simulink model "Question2"  (R2023b)
settings: Solver=VariableStepAuto  StartTime=0.0  StopTime=10.0  RelTol=1e-3
libraries: simulink x1
settings Model: Creator=joaquinsalas  LastModifiedBy=joaquinsalas

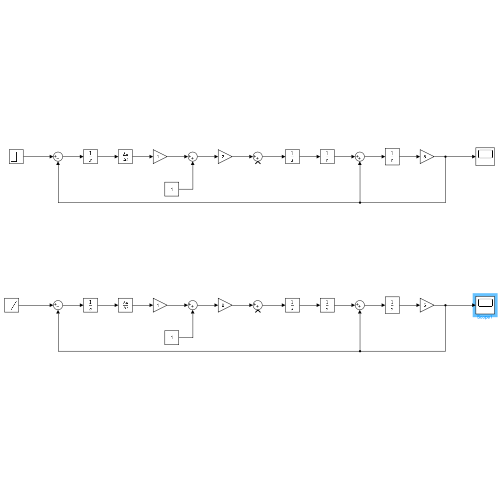
[thumbnail: Simulink's stored preview of the top-level diagram]
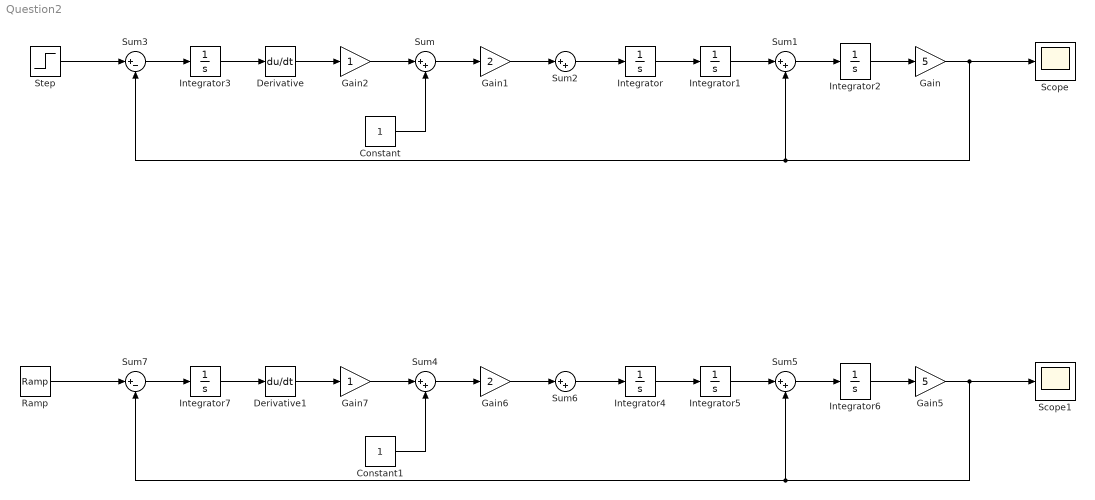
== system Question2 ==
  Constant : Constant
  Constant1 : Constant
  Derivative : Derivative
  Derivative1 : Derivative
  Gain : Gain  Gain=5
  Gain1 : Gain  Gain=2
  Gain2 : Gain
  Gain5 : Gain  Gain=5
  Gain6 : Gain  Gain=2
  Gain7 : Gain
  Integrator{,1..7} (8 alike) : Integrator
  Ramp : simulink/Sources/Ramp  slope=1  start=0  InitialOutput=0
  Scope : Scope
  Scope1 : Scope
  Step : Step  SampleTime=0
  Sum{,1..2,4..6} (6 alike) : Sum  Inputs=|++
  Sum3 : Sum  Inputs=|+-
  Sum7 : Sum  Inputs=|+-
  wires:
  Integrator/1 -> Integrator1/1
  Integrator2/1 -> Gain/1
  Integrator1/1 -> Sum1/1
  Sum1/1 -> Integrator2/1
  Integrator3/1 -> Derivative/1
  Constant/1 -> Sum/2
  Gain2/1 -> Sum/1
  Derivative/1 -> Gain2/1
  Sum/1 -> Gain1/1
  Gain1/1 -> Sum2/1
  Sum2/1 -> Integrator/1
  Sum3/1 -> Integrator3/1
  Gain/1 -> Scope/1, Sum1/2, Sum3/2
  Step/1 -> Sum3/1
  Integrator7/1 -> Derivative1/1
  Constant1/1 -> Sum4/2
  Sum4/1 -> Gain6/1
  Sum7/1 -> Integrator7/1
  Gain5/1 -> Scope1/1, Sum5/2, Sum7/2
  Gain6/1 -> Sum6/1
  Sum6/1 -> Integrator4/1
  Gain7/1 -> Sum4/1
  Integrator4/1 -> Integrator5/1
  Integrator5/1 -> Sum5/1
  Integrator6/1 -> Gain5/1
  Sum5/1 -> Integrator6/1
  Derivative1/1 -> Gain7/1
  Ramp/1 -> Sum7/1
